simulink model "Task2"  (R2020a)
settings: Solver=ode45  StartTime=0.0  StopTime=1000  RelTol=1e-3
settings Model: Creator=dvdia  LastModifiedBy=dvdia

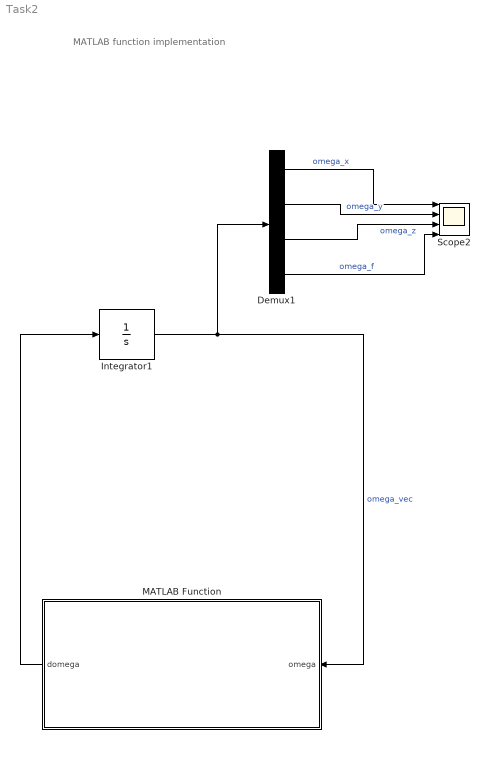
== system Task2 ==
  note: MATLAB function implementation
  Demux1 : Demux
  Integrator1 : Integrator  InitialCondition=[2*pi+1.e-6 1.e-6 1.e-6 1.e-6]
  MATLAB Function : MATLAB Function  TreatAsAtomicUnit=on
  Scope2 : Scope  NumInputPorts=4
  wires:
  Integrator1/1 -> Demux1/1, MATLAB Function/1(omega)  "omega_vec"
  Demux1/1 -> Scope2/1  "omega_x"
  MATLAB Function/1(domega) -> Integrator1/1
  Demux1/3 -> Scope2/3  "omega_z"
  Demux1/2 -> Scope2/2  "omega_y"
  Demux1/4 -> Scope2/4  "omega_f"

== matlab function Task2/MATLAB Function ==
  data: omega input; domega output
function domega = fcn(omega)

% Inertia moments

I_x = 0.07;         %  [kg*m^2]
I_y = 0.0504;       %  [kg*m^2]
I_z = 0.0109;       %  [kg*m^2]
I_r = 0.005;        %  [kg*m^2]
I_f = 0.002;

% Initial conditions

omega0_vec = [2*pi+1.e-6 1.e-6 1.e-6 1.e-6];

% Fluid damper coefficient
% c = 0.1;
c = 0.0011;
% c = 0.000001;

% Set omegas
omega_x = omega(1);
omega_y = omega(2);
omega_z = omega(3);
omega_f = omega(4);
omega_r = 2*pi;         % omega_r is constant


% Compute d_omegas
domega_f = - (c/I_f)*(omega_x + omega_f);
domega_x = ((I_y-I_z)*omega_y*omega_z - I_r * omega_r * omega_y - I_f*domega_f)/I_x;
domega_y = ((I_z-I_x)*omega_x*omega_z + I_r * omega_r * omega_x - I_f*omega_f*omega_z)/I_y;
domega_z = ((I_x - I_y)*omega_y*omega_x + I_f*omega_f*omega_y)/ I_z;


%% Output domegas
domega = [ domega_x domega_y domega_z domega_f];
end
